simulink model "Atividade_2"  (R2022a)
settings: Solver=VariableStepAuto  StartTime=0.0  StopTime=50  RelTol=1e-3
settings Model: Creator=luanv  LastModifiedBy=luanv

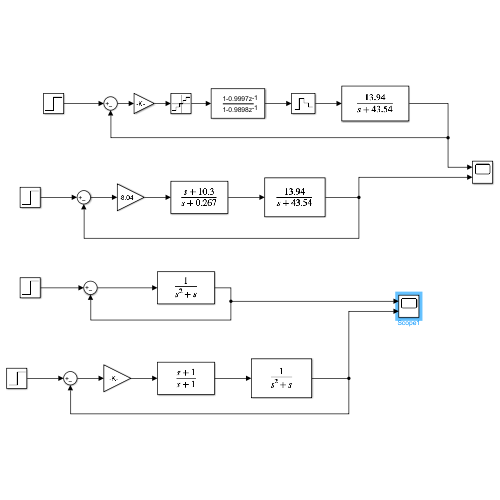
[thumbnail: Simulink's stored preview of the top-level diagram]
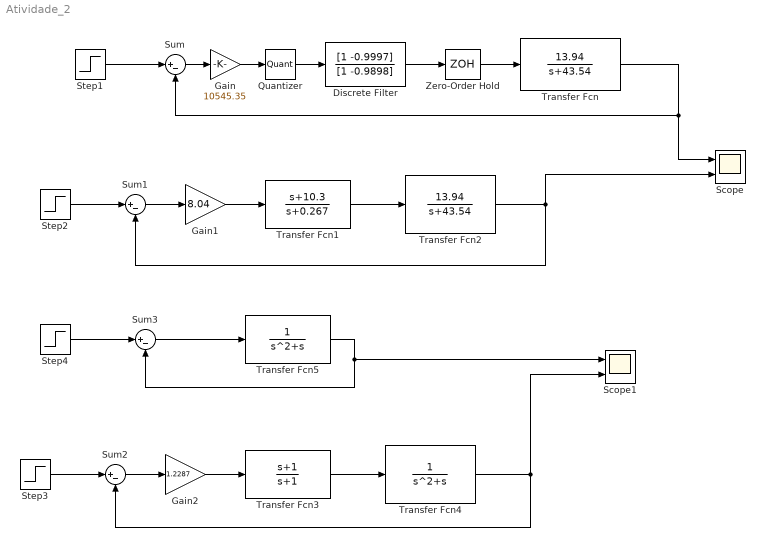
== system Atividade_2 ==
  Discrete Filter : DiscreteFilter  Numerator=[1 -0.9997]  Denominator=[1 -0.9898]  InitialStates=1
  Gain : Gain  Gain=10545.35
  Gain1 : Gain  Gain=8.04
  Gain2 : Gain  Gain=1.2287
  Quantizer : Quantizer  QuantizationInterval=0.05
  Scope : Scope  NumInputPorts=2
  Scope1 : Scope  NumInputPorts=2
  Step{1..4} (4 alike) : Step  SampleTime=0
  Sum{,1..3} (4 alike) : Sum  Inputs=|+-
  Transfer Fcn : TransferFcn  Numerator=[13.94]  Denominator=[1 43.54]
  Transfer Fcn1 : TransferFcn  Numerator=[1 10.3]  Denominator=[1 0.267]
  Transfer Fcn2 : TransferFcn  Numerator=[13.94]  Denominator=[1 43.54]
  Transfer Fcn3 : TransferFcn  Numerator=[1 1]  Denominator=[1 1]
  Transfer Fcn4 : TransferFcn  Denominator=[1 1 0]
  Transfer Fcn5 : TransferFcn  Denominator=[1 1 0]
  Zero-Order Hold : ZeroOrderHold  SampleTime=-1
  wires:
  Transfer Fcn2/1 -> Sum1/2, Scope/2
  Step2/1 -> Sum1/1
  Transfer Fcn1/1 -> Transfer Fcn2/1
  Sum1/1 -> Gain1/1
  Transfer Fcn/1 -> Scope/1, Sum/2
  Zero-Order Hold/1 -> Transfer Fcn/1
  Discrete Filter/1 -> Zero-Order Hold/1
  Step1/1 -> Sum/1
  Gain1/1 -> Transfer Fcn1/1
  Sum2/1 -> Gain2/1
  Transfer Fcn4/1 -> Scope1/2, Sum2/2
  Transfer Fcn3/1 -> Transfer Fcn4/1
  Step3/1 -> Sum2/1
  Gain2/1 -> Transfer Fcn3/1
  Step4/1 -> Sum3/1
  Sum3/1 -> Transfer Fcn5/1
  Transfer Fcn5/1 -> Sum3/2, Scope1/1
  Sum/1 -> Gain/1
  Gain/1 -> Quantizer/1
  Quantizer/1 -> Discrete Filter/1
